simulink model "Task3"  (R2024a)
settings: Solver=VariableStepAuto  StartTime=0.0  StopTime=50  RelTol=1e-3
settings Model: Creator=artemzmailov  LastModifiedBy=artemzmailov

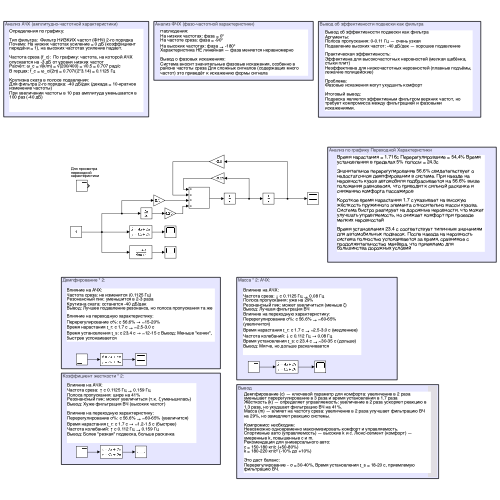
[thumbnail: Simulink's stored preview of the top-level diagram]
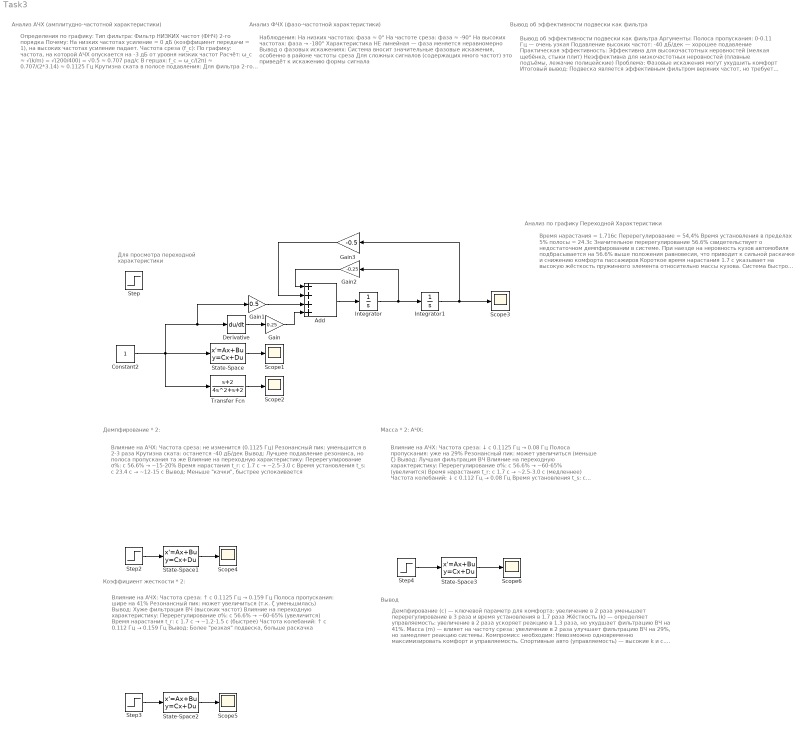
== system Task3 ==
  note: Вывод об эффективности подвески как фильтра
  note: Анализ ФЧХ (фазо-частотной характеристики)
  note: Анализ АЧХ (амплитудно-частотной характеристики)
  note: Анализ по графику Переходной Характеристики
  note: Демпфирование * 2:
  note: Влияние на АЧХ:
      | Частота среза: не изменится (0.1125 Гц)
      | Резонансный пик: уменьшится в 2-3 раза
      | Крутизна ската: останется -40 дБ/дек
      | Вывод: Лучшее подавление резонанса, но полоса пропускания та же
      |
      | Влияние на переходную характеристику:
      | Перерегулирование σ%: с 56.6% → ~15-20%
      | Время нарастания t_r: с 1.7 с → ~2.5-3.0 с
      | Время установления t_s: с 23.4 с → ~12-15 с Вывод: Меньше "качки", быстрее успокаивается
  note: Демпфирование (c) — ключевой параметр для комфорта: увеличение в 2 раза уменьшает перерегулирование в 3 раза и время установления в 1.7 раза
      | Жёсткость (k) — определяет управляемость: увеличение в 2 раза ускоряет реакцию в 1.3 раза, но ухудшает фильтрацию ВЧ на 41%.
      | Масса (m) — влияет на частоту среза: увеличение в 2 раза улучшает фильтрацию ВЧ на 29%, но замедляет реакцию системы.
      |
      | Компромисс необходим:
      | Невозможно одновременно максимизировать комфорт и управляемость.
      | Спортивные авто (управляемость) — высокие k и c. Люкс-сегмент (комфорт) — умеренные k, повышенные c и m.
      | Рекомендация для универсального авто:
      | c = 150-180 кг/с (+50-80%)
      | k = 180-220 кг/с² (-10% до +10%)
      |
      | Это даст баланс:
      | Перерегулирование - σ ≈ 30-40%, Время установления t_s ≈ 18-20 с, приемлемую фильтрацию ВЧ.
  note: Влияние на АЧХ:
      | Частота среза: ↓ с 0.1125 Гц → 0.08 Гц
      | Полоса пропускания: уже на 29%
      | Резонансный пик: может увеличиться (меньше ζ)
      | Вывод: Лучшая фильтрация ВЧ
      | Влияние на переходную характеристику:
      | Перерегулирование σ%: с 56.6% → ~60-65% (увеличится)
      | Время нарастания t_r: с 1.7 с → ~2.5-3.0 с (медленнее)
      | Частота колебаний: ↓ с 0.112 Гц → 0.08 Гц
      | Время установления t_s: с 23.4 с → ~30-35 с (дольше)
      | Вывод: Мягче, но дольше раскачивается
  note: Время нарастания = 1.716c Перерегулирование = 54,4% Время установления в пределах 5% полосы = 24.3c
      |
      | Значительное перерегулирование 56.6% свидетельствует о недостаточном демпфировании в системе. При наезде на неровность кузов автомобиля подбрасывается на 56.6% выше положения равновесия, что приводит к сильной раскачке и снижению комфорта пассажиров
      |
      | Короткое время нарастания 1.7 с указывает на высокую жёсткость пружинного элемента относительно массы кузова. Система быстро реагирует на дорожные неровности, что может улучшать управляемость, но снижает комфорт при проезде мелких неровностей
      |
      | Время установления 23.4 с соответствует типичным значениям для автомобильных подвесок. После наезда на неровность система полностью успокаивается за время, сравнимое с продолжительностью манёвра, что приемлемо для большинства дорожных условий
  note: Вывод об эффективности подвески как фильтра
      | Аргументы:
      | Полоса пропускания: 0-0.11 Гц — очень узкая
      | Подавление высоких частот: -40 дБ/дек — хорошее подавление
      |
      | Практическая эффективность:
      | Эффективна для высокочастотных неровностей (мелкая щебёнка, стыки плит)
      | Неэффективна для низкочастотных неровностей (плавные подъёмы, лежачие полицейские)
      |
      | Проблема:
      | Фазовые искажения могут ухудшить комфорт
      |
      | Итоговый вывод:
      | Подвеска является эффективным фильтром верхних частот, но требует компромисса между фильтрацией и фазовыми искажениями.
  note: Наблюдения:
      | На низких частотах: фаза ≈ 0°
      | На частоте среза: фаза ≈ -90°
      | На высоких частотах: фаза → -180°
      | Характеристика НЕ линейная — фаза меняется неравномерно
      |
      | Вывод о фазовых искажениях:
      | Система вносит значительные фазовые искажения, особенно в районе частоты среза Для сложных сигналов (содержащих много частот) это приведёт к искажению формы сигнала
  note: Для просмотра переходной характеристики
  note: Определения по графику:
      |
      | Тип фильтра: Фильтр НИЗКИХ частот (ФНЧ) 2-го порядка
      | Почему: На низких частотах усиление ≈ 0 дБ (коэффициент передачи ≈ 1), на высоких частотах усиление падает.
      |
      | Частота среза (f_c): По графику: частота, на которой АЧХ опускается на -3 дБ от уровня низких частот
      | Расчёт: ω_c ≈ √(k/m) = √(200/400) = √0.5 ≈ 0.707 рад/с
      | В герцах: f_c = ω_c/(2π) ≈ 0.707/(2*3.14) ≈ 0.1125 Гц
      |
      | Крутизна ската в полосе подавления:
      | Для фильтра 2-го порядка: -40 дБ/дек (декада = 10-кратное изменение частоты)
      | При увеличении частоты в 10 раз амплитуда уменьшается в 100 раз (-40 дБ)
  note: Влияние на АЧХ:
      | Частота среза: ↑ с 0.1125 Гц → 0.159 Гц
      | Полоса пропускания: шире на 41%
      | Резонансный пик: может увеличиться (т.к. ζ уменьшилась)
      | Вывод: Хуже фильтрация ВЧ (высоких частот)
      |
      | Влияние на переходную характеристику:
      | Перерегулирование σ%: с 56.6% → ~60-65% (увеличится)
      | Время нарастания t_r: с 1.7 с → ~1.2-1.5 с (быстрее)
      | Частота колебаний: ↑ с 0.112 Гц → 0.159 Гц
      | Вывод: Более "резкая" подвеска, больше раскачка
  note: Коэффициент жесткости * 2:
  note: Масса * 2: АЧХ:
  note: Вывод
  Add : Sum  Inputs=++++
  Constant2 : Constant
  Derivative : Derivative
  Gain : Gain  Gain=0.25
  Gain1 : Gain  Gain=0.5
  Gain2 : Gain  Gain=-0.25
  Gain3 : Gain  Gain=-0.5
  Integrator : Integrator
  Integrator1 : Integrator
  Scope{1..6} (6 alike) : Scope
  State-Space : StateSpace  A=[0 1; -0.5 -0.25]  B=[0.25; 0.4375]  C=[1, 0]  D=0  InitialCondition=0
  State-Space1 : StateSpace  A=[0 1; -0.5 -0.5]  B=[0.5; 0.4375]  C=[1, 0]  D=0  InitialCondition=0
  State-Space2 : StateSpace  A=[0 1; -1 -0.25]  B=[0.25; 0.9375]  C=[1, 0]  D=0  InitialCondition=0
  State-Space3 : StateSpace  A=[0 1; -0.25 -0.125]  B=[0.125; 0.234375]  C=[1, 0]  D=0  InitialCondition=0
  Step{,2..4} (4 alike) : Step  SampleTime=0
  Transfer Fcn : TransferFcn  Numerator=[1,2]  Denominator=[4,1,2]
  wires:
  Constant2/1 -> Transfer Fcn/1, State-Space/1, Gain1/1, Derivative/1
  Derivative/1 -> Gain/1
  Gain/1 -> Add/4
  Gain1/1 -> Add/3
  Add/1 -> Integrator/1
  Integrator1/1 -> Scope3/1, Gain3/1
  Integrator/1 -> Gain2/1, Integrator1/1
  Gain2/1 -> Add/1
  Gain3/1 -> Add/2
  State-Space/1 -> Scope1/1
  Transfer Fcn/1 -> Scope2/1
  Step3/1 -> State-Space2/1
  Step4/1 -> State-Space3/1
  Step2/1 -> State-Space1/1
  State-Space1/1 -> Scope4/1
  State-Space2/1 -> Scope5/1
  State-Space3/1 -> Scope6/1
